simulink model "ControlInteligente"  (R2017b)
settings: Solver=ode45  StartTime=0.0  StopTime=10.0  RelTol=1e-3  EnableMultiTasking=on
settings Model: Creator=Benjamin Nicolas  LastModifiedBy=Benjamin Nicolas
settings DataIOCC: LimitDataPoints=on  SaveFormat=Array
settings OptimizationCC: LifeSpan=inf
settings DebuggingCC: SFUnexpectedBacktrackingDiag=warning  SFNoUnconditionalDefaultTransitionDiag=warning  SFExecutionAtInitializationDiag=none
settings HardwareCC: ProdBitPerPointer=32  ProdBitPerSizeT=32  ProdBitPerPtrDiffT=32  ProdLargestAtomicFloat=None  ProdIntDivRoundTo=Undefined  ProdEndianess=Unspecified  ProdWordSize=32  ProdHWDeviceType=32-bit Generic
settings ModelReferenceCC: PropagateSignalLabelsOutOfModel=off
settings CodeAppCC: StateflowObjectComments=on
settings GRTTargetCC: TargetLangStandard=C89/C90 (ANSI)  GeneratePreprocessorConditionals=Disable all
settings ConfigComp: CovMetricSettings=dw  CovHtmlReporting=on  CovSaveCumulativeToWorkspaceVar=on  CovSaveSingleToWorkspaceVar=on  CovExternalEMLEnable=off

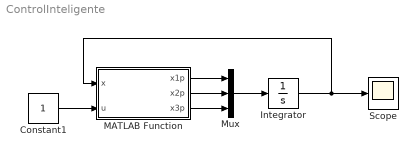
== system ControlInteligente ==
  Constant1 : Constant
  Integrator : Integrator
  MATLAB Function : MATLAB Function  TreatAsAtomicUnit=on
  Mux : Mux  Inputs=3
  Scope : Scope
  wires:
  Integrator/1 -> Scope/1, MATLAB Function/1(x)
  Constant1/1 -> MATLAB Function/2(u)
  Mux/1 -> Integrator/1
  MATLAB Function/1(x1p) -> Mux/1
  MATLAB Function/2(x2p) -> Mux/2
  MATLAB Function/3(x3p) -> Mux/3

== matlab function ControlInteligente/MATLAB Function ==
  data: x input; u input; x1p output; x2p output; x3p output
function [x1p,x2p,x3p] = SystemG(x,u)
    %Constantes
    Ra = 1.3;   m = 0.13;
    kemf = 0.7; La = 0.001;
    l = 0.2;    g = 9.81;
    %Variables
    x1 = x(1);
    x2 = x(2);
    x3 = ((m*l*g)/kemf)*sin(x(1));
    x1p = x2
    x2p = (g/l)*sin(x1)-(kemf/m*l^2)*x3
    x3p = -(Ra/La)*x3-(kemf/La)*x2+(1/La)*u
%     i= [x2;;]
